simulink model "run_gamepad"  (R2023a)
settings: Solver=VariableStepAuto  StartTime=0.0  StopTime=inf  RelTol=1e-3
libraries: aerolibanimutils x2, instrumentlib x1
settings Model: Creator=The MathWorks, Inc.  LastModifiedBy=lab5
settings SolverCC: AlgebraicLoopSolver=TrustRegion
settings DataIOCC: SaveOutput=off  SignalLogging=off  DSMLogging=off  SaveTime=off  ReturnWorkspaceOutputs=off
settings DebuggingCC: ParameterPrecisionLossMsg=none  UnconnectedInputMsg=warning  UnconnectedOutputMsg=warning  UnconnectedLineMsg=warning  ArithmeticOperatorsInVariantConditions=warning
settings ModelReferenceCC: EnableRefExpFcnMdlSchedulingChecks=on
settings SFSimCC: SimUseLocalCustomCode=off  CustomCodeUndefinedFunction=UseInterfaceOnly
settings RTWCC: RTWUseLocalCustomCode=off  DLArmComputeVersion=19.05
settings CodeAppCC: StateflowObjectComments=on

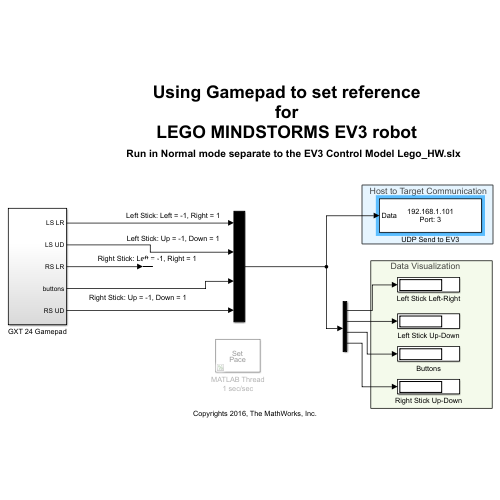
[thumbnail: Simulink's stored preview of the top-level diagram]
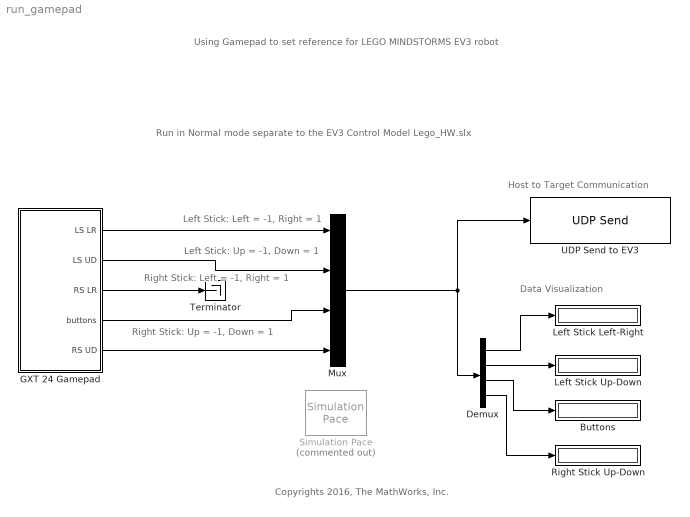
== system run_gamepad ==
  note: Copyrights 2016, The MathWorks, Inc.
  note: Using Gamepad to set reference
      | for
      | LEGO MINDSTORMS EV3 robot
  note: Data Visualization
  note: Host to Target Communication
  note: Run in Normal mode separate to the EV3 Control Model Lego_HW.slx
  note: Left Stick: Up = -1, Down = 1
  note: Left Stick: Left = -1, Right = 1
  note: Right Stick: Left = -1, Right = 1
  note: Right Stick: Up = -1, Down = 1
  Buttons : Display
  Demux : Demux
  GXT 24 Gamepad : Subsystem
  Left Stick Left-Right : Display
  Left Stick Up-Down : Display
  Mux : Mux
  Right Stick Up-Down : Display
  Simulation Pace : aerolibanimutils/Simulation Pace  Commented=on  SimulationPace=1  SleepMode=MATLAB Thread  OutputPaceError=off  SampleTime=1/30
  Terminator : Terminator
  UDP Send to EV3 : instrumentlib/UDP Send  Host=192.168.1.101  Port=3  LocalAddress=0.0.0.0  LocalPort=-1  EnablePortSharing=off  OutputDatagramPacketSize=512  ByteOrder=little-endian  EnableBlockingMode=on  SimulateUsing=Interpreted execution
  wires:
  Mux/1 -> UDP Send to EV3/1, Demux/1
  Demux/1 -> Left Stick Left-Right/1
  Demux/2 -> Left Stick Up-Down/1
  GXT 24 Gamepad/1(LS LR) -> Mux/1
  GXT 24 Gamepad/2(LS UD) -> Mux/2
  GXT 24 Gamepad/3(RS LR) -> Terminator/1
  GXT 24 Gamepad/5(RS UD) -> Mux/4
  GXT 24 Gamepad/4(buttons) -> Mux/3
  Demux/3 -> Buttons/1
  Demux/4 -> Right Stick Up-Down/1

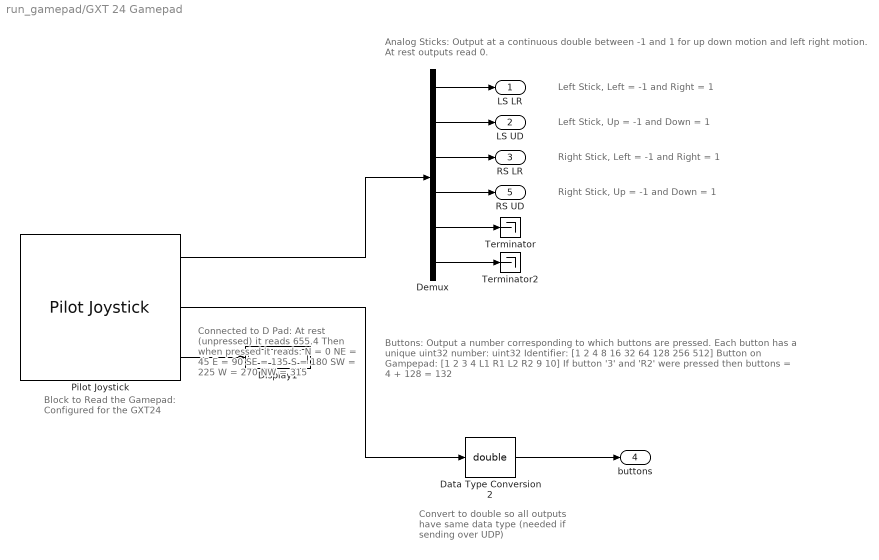
== system run_gamepad/GXT 24 Gamepad ==
  note: Analog Sticks:
      | Output at a continuous double between -1 and 1 for up down motion and left right motion. At rest outputs read 0.
  note: Connected to D Pad:
      | At rest (unpressed) it reads 655.4
      | Then when pressed it reads:
      | N = 0
      | NE = 45
      | E = 90
      | SE = 135
      | S = 180
      | SW = 225
      | W = 270
      | NW = 315
  note: Left Stick, Left = -1 and Right = 1
  note: Convert to double so all outputs have same data type
      | (needed if sending over UDP)
  note: Block to Read the Gamepad: Configured for the GXT24
  note: Left Stick, Up = -1 and Down = 1
  note: Right Stick, Left = -1 and Right = 1
  note: Right Stick, Up = -1 and Down = 1
  note: Buttons:
      | Output a number corresponding to which buttons are pressed.
      | Each button has a unique uint32 number:
      | uint32 Identifier: [1 2 4 8 16 32 64 128 256 512]
      | Button on Gampepad: [1 2 3 4 L1 R1 L2 R2 9 10]
      | If button '3' and 'R2' were pressed then buttons = 4 + 128 = 132
  Data Type Conversion2 : DataTypeConversion  OutDataTypeStr=double  RndMeth=Nearest  SaturateOnIntegerOverflow=off
  Demux : Demux  Outputs=6
  Display1 : Display
  Pilot Joystick : aerolibanimutils/Pilot Joystick  JoystickID=Joystick1  OutputConfiguration=AllOutputs  SampleTime=1/30
  Terminator : Terminator
  Terminator2 : Terminator
  LS LR : Outport  VectorParamsAs1DForOutWhenUnconnected=off
  LS UD : Outport  Port=2  VectorParamsAs1DForOutWhenUnconnected=off
  RS LR : Outport  Port=3  VectorParamsAs1DForOutWhenUnconnected=off
  buttons : Outport  Port=4  VectorParamsAs1DForOutWhenUnconnected=off
  RS UD : Outport  Port=5  VectorParamsAs1DForOutWhenUnconnected=off
  wires:
  Pilot Joystick/3 -> Display1/1
  Pilot Joystick/2 -> Data Type Conversion2/1
  Pilot Joystick/1 -> Demux/1
  Demux/1 -> LS LR/1
  Demux/2 -> LS UD/1
  Demux/3 -> RS LR/1
  Demux/4 -> RS UD/1
  Demux/6 -> Terminator2/1
  Demux/5 -> Terminator/1
  Data Type Conversion2/1 -> buttons/1
